simulink model "questao6"  (R2023a)
settings: Solver=FixedStepAuto  StartTime=0.0  StopTime=100  FixedStep=1  RelTol=1e-3
settings Model: Creator=franz  LastModifiedBy=franz

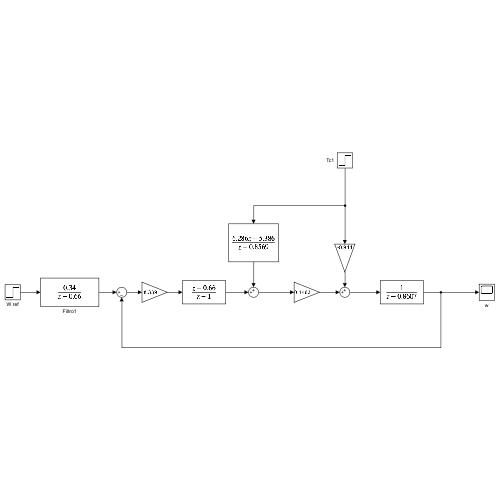
[thumbnail: Simulink's stored preview of the top-level diagram]
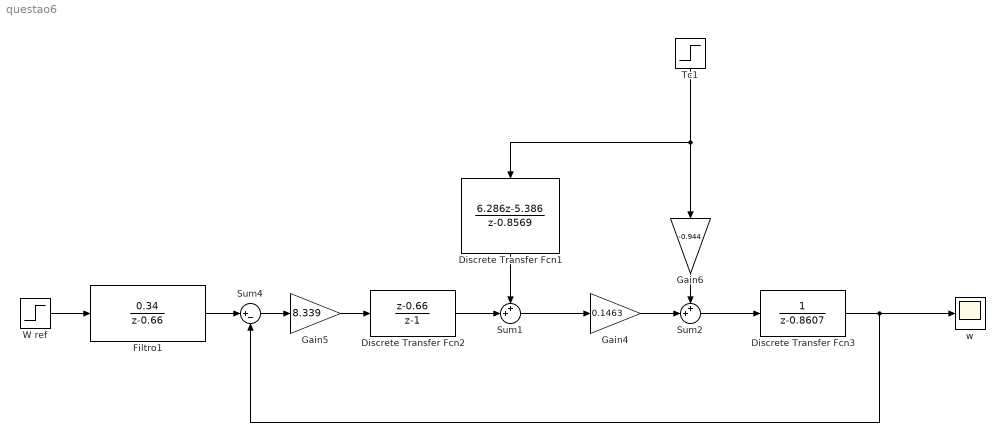
== system questao6 ==
  Discrete Transfer Fcn1 : DiscreteTransferFcn  Numerator=[6.286 -5.386]  Denominator=[1 -0.8569]
  Discrete Transfer Fcn2 : DiscreteTransferFcn  Numerator=[1 -0.66]  Denominator=[1 -1]
  Discrete Transfer Fcn3 : DiscreteTransferFcn  Numerator=[0 1]  Denominator=[1 -0.8607]
  Filtro1 : DiscreteTransferFcn  Numerator=[0 0.34]  Denominator=[1 -0.66]
  Gain4 : Gain  Gain=0.1463
  Gain5 : Gain  Gain=8.339
  Gain6 : Gain  Gain=-0.944
  Sum1 : Sum  Inputs=++|
  Sum2 : Sum  Inputs=++|
  Sum4 : Sum  Inputs=|+-
  Tc1 : Step  Time=60  Before=1  After=2  SampleTime=0
  W ref : Step  Time=10  SampleTime=0
  w : Scope
  wires:
  Filtro1/1 -> Sum4/1
  W ref/1 -> Filtro1/1
  Sum2/1 -> Discrete Transfer Fcn3/1
  Gain5/1 -> Discrete Transfer Fcn2/1
  Discrete Transfer Fcn3/1 -> Sum4/2, w/1
  Gain4/1 -> Sum2/2
  Gain6/1 -> Sum2/1
  Tc1/1 -> Discrete Transfer Fcn1/1, Gain6/1
  Sum4/1 -> Gain5/1
  Discrete Transfer Fcn2/1 -> Sum1/2
  Sum1/1 -> Gain4/1
  Discrete Transfer Fcn1/1 -> Sum1/1
